simulink model "t_t_200_tge5"  (Simulink 6.2)
settings: Solver=ode45  StartTime=0.0  StopTime=10  RelTol=1e-3
undefined symbols (not defined in the file): BEE2_usr
libraries: xbsIndex_r3 x575, xps_library x48, casper_library x20
(part 1 of 4)
settings Model: LastModifiedBy=lspitler
settings DebuggingCC: SolverPrmCheckMsg=warning

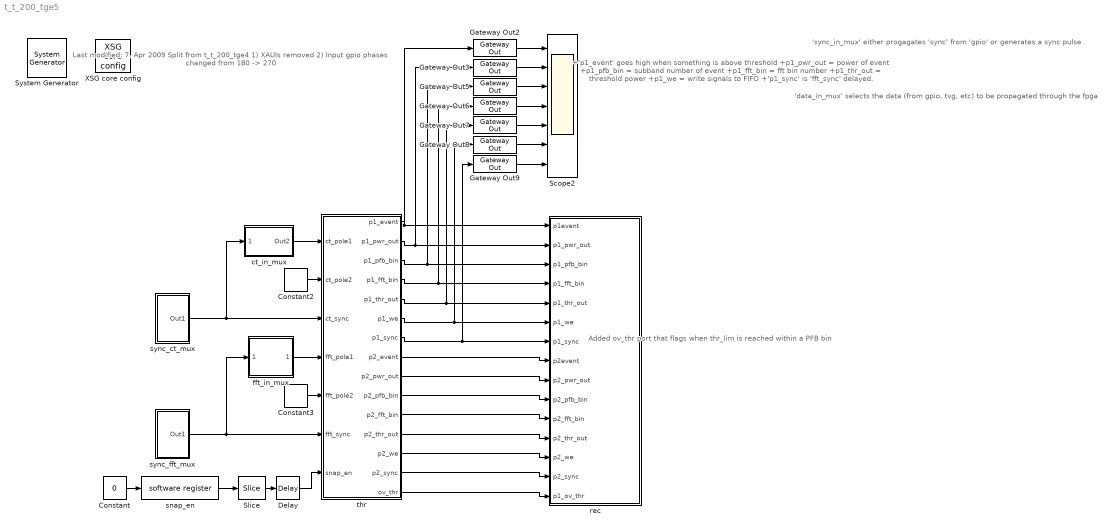
== system t_t_200_tge5 ==
  note: 'data_in_mux' selects
      | the data (from gpio, tvg, etc)
      | to be propagated
      | through the fpga
  note: 'sync_in_mux' either
      | progagates 'sync' from 'gpio'
      | or generates a sync pulse
  note: Last modified: 7. Apr 2009
      | Split from t_t_200_tge4
      | 1) XAUIs removed
      | 2) Input gpio phases changed
      | from 180 -> 270
  note: +'p1_event' goes high when something is above threshold
      | +p1_pwr_out = power of event
      | +p1_pfb_bin = subband number of event
      | +p1_fft_bin = fft bin number
      | +p1_thr_out = threshold power
      | +p1_we = write signals to FIFO
      | +'p1_sync' is 'fft_sync' delayed.
  note: Added ov_thr port that
      | flags when thr_lim is reached
      | within a PFB  bin
  " System Generator" : xbsIndex_r3/ System Generator  Tag=genX  xilinxfamily=Virtex2P  part=xc2vp70  speed=-7  package=ff1704  synthesis_tool=XST  directory=./t_t_200_tge5/sysgen  testbench=off  simulink_period=1  sysclk_period=5  incr_netlist=off  trim_vbits=Everywhere in SubSystem  dbl_ovrd=According to Block Masks  core_generation=According to Block Masks  run_coregen=off  deprecated_control=off  eval_field=0
      settings: AttributesFormatString=System\nGenerator
  Constant : Constant  Value=0
  Constant2 : xbsIndex_r3/Constant  const=0  equ=P=C  arith_type=Unsigned  n_bits=36  bin_pt=0  opselect=C  inp2=PCIN>>17  opr=+  inp1=P  carry=CIN  iostate=0  explicit_period=on  period=1  dbl_ovrd=off
  Constant3 : xbsIndex_r3/Constant  const=0  equ=P=C  arith_type=Unsigned  n_bits=36  bin_pt=0  opselect=C  inp2=PCIN>>17  opr=+  inp1=P  carry=CIN  iostate=0  explicit_period=on  period=1  dbl_ovrd=off
  Delay : xbsIndex_r3/Delay  latency=1  reg_retiming=on  explicit_period=off  period=1  en=off  accept_only_valid=off  init_zero=on  dbl_ovrd=off  show_param=off
      settings: xl_area=[0, 0, 0, 0, 0, 0, 0]
  Gateway Out{2..3,5..9} (7 alike) : xbsIndex_r3/Gateway Out  output_type=Double  nbits=8  bin_pt=6  arith_type=Boolean  quantization=Truncate  overflow=Wrap  hdl_port=on  timing_constraint=None  locs_specified=off  LOCs={}  needs_fixed_name=off  show_param=off
      settings: xl_area=[0, 0, 0, 0, 0, 0, 0]
  Scope2 : Scope  NumInputPorts=7
      settings: YMin=0.95~1.71474~-1~200~-1~0~-1  YMax=1.05~1.89524~1~900~1~1~1  SaveName=ScopeData21
  Slice : xbsIndex_r3/Slice  mode=Lower Bit Location + Width  nbits=1  bit1=0  base1=MSB of Input  bit0=0  base0=LSB of Input  boolean_output=on  explicit_period=off  period=1  dbl_ovrd=off
  XSG core config : xps_library/XSG core config  Tag=xps:xsg  hw_sys=BEE2_usr  ibob_linux=off  clk_src=usr_clk2x  gpio_clk_io_group=iBOB:sma  gpio_clk_bit_index=0  clk_rate=200  sample_period=1  synthesis_tool=XST  mpc_type=powerpc405
  ct_in_mux : Subsystem  mask{data_sel=3}
      mask prompts: data_sel "Data mux (0 = previous fpga, 1 = ones, 2 = zeros, 3 = tvg)"
  fft_in_mux : Subsystem  mask{data_sel=1}
      mask prompts: data_sel "Data mux (0 = previous fpga, 1 = tvg)"
  rec : Subsystem  mask{PFBSize=12, FFTSize=15, CPUWidth=32}
      mask prompts: PFBSize "PFB Size (2^?)"; FFTSize "FFT Size (2^?)"; CPUWidth "CPU Word Size"
  snap_en : xps_library/software register  Tag=xps:sw_reg  io_dir=From Processor  arith_type=Unsigned  bitwidth=32  bin_pt=0  sample_period=1  gw_name=t_t_200_tge5_snap_en_user_data_out
  sync_ct_mux : Subsystem  mask{sync_sel=1, sync_period=(2^18)-2}
      mask prompts: sync_sel "Sync Mux (0 = from previous FPGA, 1 = simulated sync)"; sync_period "Simulated sync period(number of clock cycles)"
  sync_fft_mux : Subsystem  mask{sync_sel=1, sync_period=(2^15)-2}
      mask prompts: sync_sel "Sync Mux (0 = from previous FPGA, 1 = simulated sync)"; sync_period "Simulated sync period(number of clock cycles)"
  thr : Subsystem  mask{PFBSize=12, FFTSize=15, DataWidth=18, CPUWidth=32}
      mask prompts: PFBSize "PFB Size (2^?)"; FFTSize "FFT Size (2^?)"; DataWidth "Data Bitwidth"; CPUWidth "CPU Word Size"
  wires:
  sync_ct_mux/1(Out1) -> ct_in_mux/1(trig_in), thr/3(ct_sync)
  Constant2/1 -> thr/2(ct_pole2)
  Constant3/1 -> thr/5(fft_pole2)
  thr/2(p1_pwr_out) -> Gateway Out3/1, rec/2(p1_pwr_out)
  thr/3(p1_pfb_bin) -> Gateway Out5/1, rec/3(p1_pfb_bin)
  thr/4(p1_fft_bin) -> Gateway Out6/1, rec/4(p1_fft_bin)
  thr/5(p1_thr_out) -> Gateway Out7/1, rec/5(p1_thr_out)
  thr/1(p1_event) -> Gateway Out2/1, rec/1(p1event)
  Gateway Out2/1 -> Scope2/1
  Gateway Out3/1 -> Scope2/2
  Gateway Out5/1 -> Scope2/3
  Gateway Out6/1 -> Scope2/4
  Gateway Out7/1 -> Scope2/5
  Gateway Out8/1 -> Scope2/6
  Gateway Out9/1 -> Scope2/7
  thr/6(p1_we) -> Gateway Out8/1, rec/6(p1_we)
  thr/7(p1_sync) -> Gateway Out9/1, rec/7(p1_sync)
  Constant/1 -> snap_en/1
  snap_en/1 -> Slice/1
  Slice/1 -> Delay/1
  thr/8(p2_event) -> rec/8(p2event)
  thr/9(p2_pwr_out) -> rec/9(p2_pwr_out)
  thr/10(p2_pfb_bin) -> rec/10(p2_pfb_bin)
  thr/11(p2_fft_bin) -> rec/11(p2_fft_bin)
  thr/12(p2_thr_out) -> rec/12(p2_thr_out)
  thr/13(p2_we) -> rec/13(p2_we)
  thr/14(p2_sync) -> rec/14(p2_sync)
  thr/15(ov_thr) -> rec/15(p1_ov_thr)
  sync_fft_mux/1(Out1) -> fft_in_mux/1(trig_in), thr/6(fft_sync)
  ct_in_mux/1(Out2) -> thr/1(ct_pole1)
  fft_in_mux/1(Out2) -> thr/4(fft_pole1)
  Delay/1 -> thr/7("snap_en ")

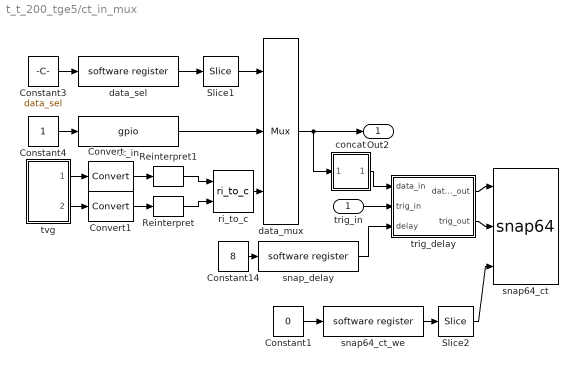
== system t_t_200_tge5/ct_in_mux ==
  trig_in : Inport  Port=1  LatchInput=off
  Constant1 : Constant  Value=0
  Constant14 : Constant  Value=8
  Constant3 : Constant  Value=data_sel
  Constant4 : Constant
  Convert : xbsIndex_r3/Convert  arith_type=Unsigned  n_bits=18  bin_pt=0  quantization=Truncate  overflow=Wrap  latency=0  explicit_period=on  period=1  dbl_ovrd=off  show_param=off  inserted_by_tool=off  pipeline=off
      settings: xl_area=[0, 0, 0, 0, 0, 0, 0]
  Convert1 : xbsIndex_r3/Convert  arith_type=Unsigned  n_bits=18  bin_pt=0  quantization=Truncate  overflow=Wrap  latency=0  explicit_period=on  period=1  dbl_ovrd=off  show_param=off  inserted_by_tool=off  pipeline=off
      settings: xl_area=[0, 0, 0, 0, 0, 0, 0]
  Reinterpret : xbsIndex_r3/Reinterpret  force_arith_type=on  arith_type="Signed  (2's comp)"  force_bin_pt=on  bin_pt=17  force_valid=on
  Reinterpret1 : xbsIndex_r3/Reinterpret  force_arith_type=on  arith_type="Signed  (2's comp)"  force_bin_pt=on  bin_pt=17  force_valid=on
  Slice1 : xbsIndex_r3/Slice  mode=Lower Bit Location + Width  nbits=1  bit1=0  base1=MSB of Input  bit0=0  base0=LSB of Input  boolean_output=off  explicit_period=off  period=1  dbl_ovrd=off
  Slice2 : xbsIndex_r3/Slice  mode=Lower Bit Location + Width  nbits=1  bit1=0  base1=MSB of Input  bit0=0  base0=LSB of Input  boolean_output=on  explicit_period=off  period=1  dbl_ovrd=off
  concat : Subsystem
  ct_in : xps_library/gpio  Tag=xps:gpio  io_group=BEE2_usr:rightlink  io_dir=in  arith_type=Unsigned  bitwidth=36  bin_pt=0  bit_index=[0:35]  sample_period=1  use_single_ended=off  use_ddr=off  reg_iob=on  reg_clk_phase=270  termination=None
  data_mux : xbsIndex_r3/Mux  inputs=2  precision=Full  arith_type="Signed  (2's comp)"  n_bits=8  bin_pt=2  quantization=Truncate  overflow=Wrap  latency=2  explicit_period=on  period=1  en=off  dbl_ovrd=off  show_param=off  mux_type=off  use_rpm=off  gen_core=off
      settings: xl_area=[0, 0, 0, 0, 0, 0, 0]
  data_sel : xps_library/software register  Tag=xps:sw_reg  io_dir=From Processor  arith_type=Unsigned  bitwidth=32  bin_pt=0  sample_period=1  gw_name=t_t_200_tge5_ct_in_mux_data_sel_user_data_out
  ri_to_c : casper_library/Misc/ri_to_c
  snap64_ct : casper_library/Scopes/snap64  nsamples=11
  snap64_ct_we : xps_library/software register  Tag=xps:sw_reg  io_dir=From Processor  arith_type=Unsigned  bitwidth=32  bin_pt=0  sample_period=1  gw_name=t_t_200_tge5_ct_in_mux_snap64_ct_we_user_data_out
  snap_delay : xps_library/software register  Tag=xps:sw_reg  io_dir=From Processor  arith_type=Unsigned  bitwidth=32  bin_pt=0  sample_period=1  gw_name=t_t_200_tge5_ct_in_mux_snap_delay_user_data_out
  trig_delay : Subsystem
  tvg : Subsystem
  Out2 : Outport
  wires:
  data_sel/1 -> Slice1/1
  Constant3/1 -> data_sel/1
  Slice1/1 -> data_mux/1
  ct_in/1 -> data_mux/2
  Constant4/1 -> ct_in/1
  data_mux/1 -> Out2/1, concat/1(In1)
  ri_to_c/1 -> data_mux/3
  Convert/1 -> Reinterpret1/1
  Convert1/1 -> Reinterpret/1
  Reinterpret1/1 -> ri_to_c/1
  Reinterpret/1 -> ri_to_c/2
  tvg/1(re_out) -> Convert/1
  tvg/2(im_out) -> Convert1/1
  Constant1/1 -> snap64_ct_we/1
  snap64_ct_we/1 -> Slice2/1
  Slice2/1 -> snap64_ct/3
  Constant14/1 -> snap_delay/1
  snap_delay/1 -> trig_delay/3(delay)
  trig_delay/1(data_out) -> snap64_ct/1
  trig_delay/2(trig_out) -> snap64_ct/2
  concat/1(Out1) -> trig_delay/1(data_in)
  trig_in/1 -> trig_delay/2(trig_in)

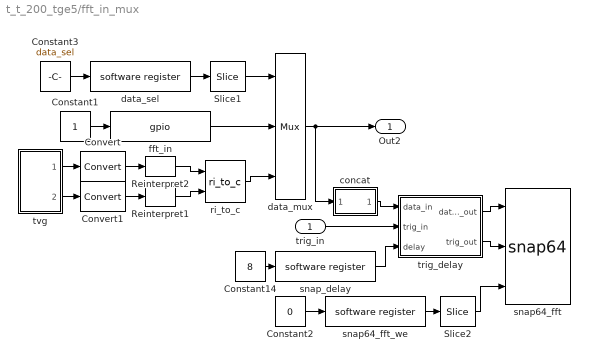
== system t_t_200_tge5/fft_in_mux ==
  trig_in : Inport  Port=1  LatchInput=off
  Constant1 : Constant
  Constant14 : Constant  Value=8
  Constant2 : Constant  Value=0
  Constant3 : Constant  Value=data_sel
  Convert : xbsIndex_r3/Convert  arith_type=Unsigned  n_bits=18  bin_pt=0  quantization=Truncate  overflow=Wrap  latency=0  explicit_period=on  period=1  dbl_ovrd=off  show_param=off  inserted_by_tool=off  pipeline=off
      settings: xl_area=[0, 0, 0, 0, 0, 0, 0]
  Convert1 : xbsIndex_r3/Convert  arith_type=Unsigned  n_bits=18  bin_pt=0  quantization=Truncate  overflow=Wrap  latency=0  explicit_period=on  period=1  dbl_ovrd=off  show_param=off  inserted_by_tool=off  pipeline=off
      settings: xl_area=[0, 0, 0, 0, 0, 0, 0]
  Reinterpret1 : xbsIndex_r3/Reinterpret  force_arith_type=on  arith_type="Signed  (2's comp)"  force_bin_pt=on  bin_pt=17  force_valid=on
  Reinterpret2 : xbsIndex_r3/Reinterpret  force_arith_type=on  arith_type="Signed  (2's comp)"  force_bin_pt=on  bin_pt=17  force_valid=on
  Slice1 : xbsIndex_r3/Slice  mode=Lower Bit Location + Width  nbits=1  bit1=0  base1=MSB of Input  bit0=0  base0=LSB of Input  boolean_output=off  explicit_period=off  period=1  dbl_ovrd=off
  Slice2 : xbsIndex_r3/Slice  mode=Lower Bit Location + Width  nbits=1  bit1=0  base1=MSB of Input  bit0=0  base0=LSB of Input  boolean_output=on  explicit_period=off  period=1  dbl_ovrd=off
  concat : Subsystem
  data_mux : xbsIndex_r3/Mux  inputs=2  precision=Full  arith_type="Signed  (2's comp)"  n_bits=8  bin_pt=2  quantization=Truncate  overflow=Wrap  latency=2  explicit_period=on  period=1  en=off  dbl_ovrd=off  show_param=off  mux_type=off  use_rpm=off  gen_core=off
      settings: xl_area=[0, 0, 0, 0, 0, 0, 0]
  data_sel : xps_library/software register  Tag=xps:sw_reg  io_dir=From Processor  arith_type=Unsigned  bitwidth=32  bin_pt=0  sample_period=1  gw_name=t_t_200_tge5_fft_in_mux_data_sel_user_data_out
  fft_in : xps_library/gpio  Tag=xps:gpio  io_group=BEE2_usr:rightlink  io_dir=in  arith_type=Unsigned  bitwidth=36  bin_pt=0  bit_index=[37:72]  sample_period=1  use_single_ended=off  use_ddr=off  reg_iob=on  reg_clk_phase=270  termination=None
  ri_to_c : casper_library/Misc/ri_to_c
  snap64_fft : casper_library/Scopes/snap64  nsamples=11
  snap64_fft_we : xps_library/software register  Tag=xps:sw_reg  io_dir=From Processor  arith_type=Unsigned  bitwidth=32  bin_pt=0  sample_period=1  gw_name=t_t_200_tge5_fft_in_mux_snap64_fft_we_user_data_out
  snap_delay : xps_library/software register  Tag=xps:sw_reg  io_dir=From Processor  arith_type=Unsigned  bitwidth=32  bin_pt=0  sample_period=1  gw_name=t_t_200_tge5_fft_in_mux_snap_delay_user_data_out
  trig_delay : Subsystem
  tvg : Subsystem
  Out2 : Outport
  wires:
  data_sel/1 -> Slice1/1
  Constant3/1 -> data_sel/1
  Slice1/1 -> data_mux/1
  fft_in/1 -> data_mux/2
  Constant1/1 -> fft_in/1
  data_mux/1 -> Out2/1, concat/1(In1)
  Convert1/1 -> Reinterpret1/1
  Reinterpret1/1 -> ri_to_c/2
  tvg/2(im_out) -> Convert1/1
  tvg/1(re_out) -> Convert/1
  Convert/1 -> Reinterpret2/1
  Reinterpret2/1 -> ri_to_c/1
  ri_to_c/1 -> data_mux/3
  Constant2/1 -> snap64_fft_we/1
  snap64_fft_we/1 -> Slice2/1
  Slice2/1 -> snap64_fft/3
  Constant14/1 -> snap_delay/1
  snap_delay/1 -> trig_delay/3(delay)
  trig_delay/1(data_out) -> snap64_fft/1
  trig_delay/2(trig_out) -> snap64_fft/2
  concat/1(Out1) -> trig_delay/1(data_in)
  trig_in/1 -> trig_delay/2(trig_in)

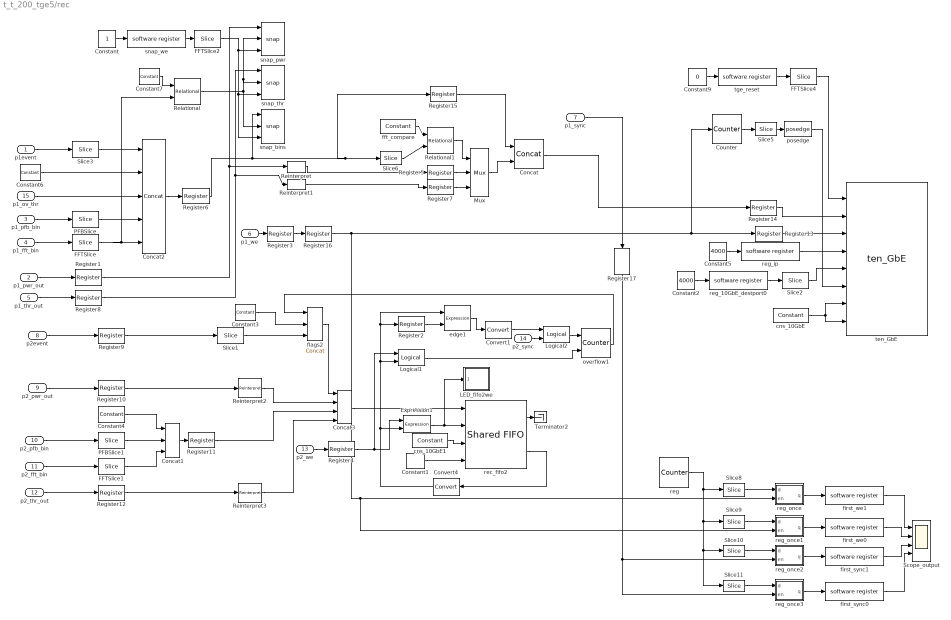
== system t_t_200_tge5/rec ==
  p1event : Inport  Port=1  LatchInput=off
  p1_pwr_out : Inport  Port=2  LatchInput=off
  p1_pfb_bin : Inport  Port=3  LatchInput=off
  p1_fft_bin : Inport  Port=4  LatchInput=off
  p1_thr_out : Inport  Port=5  LatchInput=off
  p1_we : Inport  Port=6  LatchInput=off
  p1_sync : Inport  Port=7  LatchInput=off
  p2event : Inport  Port=8  LatchInput=off
  p2_pwr_out : Inport  Port=9  LatchInput=off
  p2_pfb_bin : Inport  Port=10  LatchInput=off
  p2_fft_bin : Inport  Port=11  LatchInput=off
  p2_thr_out : Inport  Port=12  LatchInput=off
  p2_we : Inport  Port=13  LatchInput=off
  p2_sync : Inport  Port=14  LatchInput=off
  p1_ov_thr : Inport  Port=15  LatchInput=off
  Concat : xbsIndex_r3/Concat  num_inputs=2  explicit_period=off  period=1  dbl_ovrd=off
  Concat1 : xbsIndex_r3/Concat  num_inputs=3  explicit_period=off  period=1  dbl_ovrd=off
  Concat2 : xbsIndex_r3/Concat  num_inputs=5  explicit_period=on  period=1  dbl_ovrd=off
  Concat3 : xbsIndex_r3/Concat  num_inputs=4  explicit_period=off  period=1  dbl_ovrd=off
  Constant : Constant
  Constant1 : xbsIndex_r3/Constant  const=512-4  equ=P=C  arith_type=Unsigned  n_bits=32  bin_pt=0  opselect=C  inp2=PCIN>>17  opr=+  inp1=P  carry=CIN  iostate=0  explicit_period=on  period=1  dbl_ovrd=off
  Constant2 : Constant  Value=4000
  Constant3 : xbsIndex_r3/Constant  const=0  equ=P=C  arith_type=Unsigned  n_bits=15  bin_pt=0  opselect=C  inp2=PCIN>>17  opr=+  inp1=P  carry=CIN  iostate=0  explicit_period=on  period=1  dbl_ovrd=off
  Constant4 : xbsIndex_r3/Constant  const=0  equ=P=C  arith_type=Unsigned  n_bits=CPUWidth-PFBSize-FFTSize  bin_pt=0  opselect=C  inp2=PCIN>>17  opr=+  inp1=P  carry=CIN  iostate=0  explicit_period=on  period=1  dbl_ovrd=off
  Constant5 : Constant  Value=4000
  Constant6 : xbsIndex_r3/Constant  const=0  equ=P=C  arith_type=Unsigned  n_bits=3  bin_pt=0  opselect=C  inp2=PCIN>>17  opr=+  inp1=P  carry=CIN  iostate=0  explicit_period=on  period=1  dbl_ovrd=off
  Constant7 : xbsIndex_r3/Constant  const=0  equ=P=C  arith_type=Unsigned  n_bits=15  bin_pt=0  opselect=C  inp2=PCIN>>17  opr=+  inp1=P  carry=CIN  iostate=0  explicit_period=on  period=1  dbl_ovrd=off
  Constant9 : Constant  Value=0
  Convert1 : xbsIndex_r3/Convert  arith_type=Boolean  n_bits=8  bin_pt=6  quantization=Truncate  overflow=Wrap  latency=0  explicit_period=off  period=1  dbl_ovrd=off  show_param=off  inserted_by_tool=off  pipeline=off
      settings: xl_area=[0, 0, 0, 0, 0, 0, 0]
  Convert4 : xbsIndex_r3/Convert  Orientation=left  arith_type=Boolean  n_bits=8  bin_pt=6  quantization=Truncate  overflow=Wrap  latency=0  explicit_period=off  period=1  dbl_ovrd=off  show_param=off  inserted_by_tool=off  pipeline=off
      settings: xl_area=[0, 0, 0, 0, 0, 0, 0]
  Counter : xbsIndex_r3/Counter  cnt_type=Free Running  n_bits=9  bin_pt=0  arith_type=Unsigned  start_count=0  cnt_to=Inf  cnt_by_val=1  operation=Up  explicit_period=off  period=1  load_pin=off  rst=off  en=on  dbl_ovrd=off  show_param=off  use_rpm=on  gen_core=off
      settings: xl_area=[0, 0, 0, 0, 0, 0, 0]
  Expression1 : xbsIndex_r3/Expression  expression=a & ~b  precision=Full  arith_type=Unsigned  n_bits=8  bin_pt=2  align_bp=on  latency=0  explicit_period=off  period=1  en=off  dbl_ovrd=off  show_param=off
      settings: xl_area=[0, 0, 0, 0, 0, 0, 0]
  FFTSlice : xbsIndex_r3/Slice  mode=Lower Bit Location + Width  nbits=FFTSize  bit1=0  base1=MSB of Input  bit0=0  base0=LSB of Input  boolean_output=off  explicit_period=off  period=1  dbl_ovrd=off
  FFTSlice1 : xbsIndex_r3/Slice  mode=Lower Bit Location + Width  nbits=FFTSize  bit1=0  base1=MSB of Input  bit0=0  base0=LSB of Input  boolean_output=off  explicit_period=off  period=1  dbl_ovrd=off
  FFTSlice2 : xbsIndex_r3/Slice  mode=Lower Bit Location + Width  nbits=1  bit1=0  base1=MSB of Input  bit0=0  base0=LSB of Input  boolean_output=on  explicit_period=off  period=1  dbl_ovrd=off
  FFTSlice4 : xbsIndex_r3/Slice  mode=Lower Bit Location + Width  nbits=1  bit1=0  base1=MSB of Input  bit0=0  base0=LSB of Input  boolean_output=on  explicit_period=off  period=1  dbl_ovrd=off
  LED_fifo2we : Subsystem  mask{pulse_length=200000}
      mask prompts: pulse_length "Pulse Length (samples)"
  Logical1 : xbsIndex_r3/Logical  logical_function=AND  inputs=2  precision=Full  arith_type=Unsigned  n_bits=8  bin_pt=2  align_bp=on  latency=0  explicit_period=off  period=1  en=off  dbl_ovrd=off  show_param=off
      settings: xl_area=[0, 0, 0, 0, 0, 0, 0]
  Logical2 : xbsIndex_r3/Logical  logical_function=OR  inputs=2  precision=Full  arith_type=Unsigned  n_bits=8  bin_pt=2  align_bp=on  latency=0  explicit_period=off  period=1  en=off  dbl_ovrd=off  show_param=off
      settings: xl_area=[0, 0, 0, 0, 0, 0, 0]
  Mux : xbsIndex_r3/Mux  inputs=2  precision=Full  arith_type="Signed  (2's comp)"  n_bits=8  bin_pt=2  quantization=Truncate  overflow=Wrap  latency=0  explicit_period=off  period=1  en=off  dbl_ovrd=off  show_param=off  mux_type=off  use_rpm=off  gen_core=off
      settings: xl_area=[0, 0, 0, 0, 0, 0, 0]
  PFBSlice : xbsIndex_r3/Slice  mode=Lower Bit Location + Width  nbits=PFBSize  bit1=0  base1=MSB of Input  bit0=0  base0=LSB of Input  boolean_output=off  explicit_period=off  period=1  dbl_ovrd=off
  PFBSlice1 : xbsIndex_r3/Slice  mode=Lower Bit Location + Width  nbits=PFBSize  bit1=0  base1=MSB of Input  bit0=0  base0=LSB of Input  boolean_output=off  explicit_period=off  period=1  dbl_ovrd=off
  Register{1..16} (16 alike) : xbsIndex_r3/Register  init=0  reg_only_valid=off  explicit_period=on  period=1  rst=off  en=off  out_en=off  dbl_ovrd=off  show_param=off
      settings: xl_area=[0, 0, 0, 0, 0, 0, 0]
  Register17 : xbsIndex_r3/Register  Orientation=down  init=0  reg_only_valid=off  explicit_period=on  period=1  rst=off  en=off  out_en=off  dbl_ovrd=off  show_param=off
      settings: xl_area=[0, 0, 0, 0, 0, 0, 0]
  Reinterpret{,1..3} (4 alike) : xbsIndex_r3/Reinterpret  force_arith_type=on  arith_type=Unsigned  force_bin_pt=on  bin_pt=0  force_valid=on
  Relational : xbsIndex_r3/Relational  mode=a=b  latency=1  explicit_period=off  period=1  en=off  dbl_ovrd=off  show_param=off
      settings: xl_area=[0, 0, 0, 0, 0, 0, 0]
  Relational1 : xbsIndex_r3/Relational  mode=a=b  latency=1  explicit_period=off  period=1  en=off  dbl_ovrd=off  show_param=off
      settings: xl_area=[0, 0, 0, 0, 0, 0, 0]
  Scope_output : Scope  NumInputPorts=4
      settings: TimeRange=1  YMin=502.55~502.55~500.65~500.65  YMax=555.45~555.45~553.35~553.35  SaveName=ScopeData5
  Slice1 : xbsIndex_r3/Slice  mode=Lower Bit Location + Width  nbits=1  bit1=0  base1=MSB of Input  bit0=0  base0=LSB of Input  boolean_output=off  explicit_period=off  period=1  dbl_ovrd=off
  Slice10 : xbsIndex_r3/Slice  mode=Upper Bit Location + Width  nbits=32  bit1=0  base1=MSB of Input  bit0=0  base0=LSB of Input  boolean_output=off  explicit_period=off  period=1  dbl_ovrd=off
  Slice11 : xbsIndex_r3/Slice  mode=Lower Bit Location + Width  nbits=32  bit1=-3  base1=MSB of Input  bit0=0  base0=LSB of Input  boolean_output=off  explicit_period=off  period=1  dbl_ovrd=off
  Slice2 : xbsIndex_r3/Slice  mode=Lower Bit Location + Width  nbits=16  bit1=0  base1=MSB of Input  bit0=0  base0=LSB of Input  boolean_output=off  explicit_period=off  period=1  dbl_ovrd=off
  Slice3 : xbsIndex_r3/Slice  mode=Lower Bit Location + Width  nbits=1  bit1=0  base1=MSB of Input  bit0=0  base0=LSB of Input  boolean_output=off  explicit_period=off  period=1  dbl_ovrd=off
  Slice5 : xbsIndex_r3/Slice  mode=Upper Bit Location + Width  nbits=1  bit1=0  base1=MSB of Input  bit0=64  base0=LSB of Input  boolean_output=on  explicit_period=off  period=1  dbl_ovrd=off
  Slice6 : xbsIndex_r3/Slice  mode=Lower Bit Location + Width  nbits=15  bit1=0  base1=MSB of Input  bit0=0  base0=LSB of Input  boolean_output=off  explicit_period=off  period=1  dbl_ovrd=off
  Slice8 : xbsIndex_r3/Slice  mode=Upper Bit Location + Width  nbits=32  bit1=0  base1=MSB of Input  bit0=0  base0=LSB of Input  boolean_output=off  explicit_period=off  period=1  dbl_ovrd=off
  Slice9 : xbsIndex_r3/Slice  mode=Lower Bit Location + Width  nbits=32  bit1=-3  base1=MSB of Input  bit0=0  base0=LSB of Input  boolean_output=off  explicit_period=off  period=1  dbl_ovrd=off
  Terminator2 : Terminator
  cns_10GbE : xbsIndex_r3/Constant  const=0  equ=P=C  arith_type=Boolean  n_bits=32  bin_pt=0  opselect=C  inp2=PCIN>>17  opr=+  inp1=P  carry=CIN  iostate=0  explicit_period=on  period=1  dbl_ovrd=off
  cns_10GbE1 : xbsIndex_r3/Constant  const=0  equ=P=C  arith_type=Boolean  n_bits=32  bin_pt=0  opselect=C  inp2=PCIN>>17  opr=+  inp1=P  carry=CIN  iostate=0  explicit_period=on  period=1  dbl_ovrd=off
  edge1 : xbsIndex_r3/Expression  expression=a & ~b  precision=Full  arith_type=Unsigned  n_bits=8  bin_pt=2  align_bp=on  latency=0  explicit_period=off  period=1  en=off  dbl_ovrd=off  show_param=off
      settings: xl_area=[0, 0, 0, 0, 0, 0, 0]
  fft_compare : xbsIndex_r3/Constant  const=0  equ=P=C  arith_type=Unsigned  n_bits=15  bin_pt=0  opselect=C  inp2=PCIN>>17  opr=+  inp1=P  carry=CIN  iostate=0  explicit_period=on  period=1  dbl_ovrd=off
  first_sync0 : xps_library/software register  Tag=xps:sw_reg  io_dir=To Processor  arith_type=Unsigned  bitwidth=32  bin_pt=0  sample_period=1  gw_name=t_t_200_tge5_rec_first_sync0_user_data_in
  first_sync1 : xps_library/software register  Tag=xps:sw_reg  io_dir=To Processor  arith_type=Unsigned  bitwidth=32  bin_pt=0  sample_period=1  gw_name=t_t_200_tge5_rec_first_sync1_user_data_in
  first_we0 : xps_library/software register  Tag=xps:sw_reg  io_dir=To Processor  arith_type=Unsigned  bitwidth=32  bin_pt=0  sample_period=1  gw_name=t_t_200_tge5_rec_first_we0_user_data_in
  first_we1 : xps_library/software register  Tag=xps:sw_reg  io_dir=To Processor  arith_type=Unsigned  bitwidth=32  bin_pt=0  sample_period=1  gw_name=t_t_200_tge5_rec_first_we1_user_data_in
  flags2 : xbsIndex_r3/Concat  num_inputs=3  explicit_period=off  period=1  dbl_ovrd=off
  overflow1 : xbsIndex_r3/Counter  cnt_type=Count Limited  n_bits=16  bin_pt=0  arith_type=Unsigned  start_count=0  cnt_to=Inf  cnt_by_val=1  operation=Up  explicit_period=off  period=1  load_pin=off  rst=on  en=on  dbl_ovrd=off  show_param=off  use_rpm=on  gen_core=off
      settings: xl_area=[0, 0, 0, 0, 0, 0, 0]
  posedge : casper_library/Misc/posedge  Tag=Rising Edge Detector
  rec_fifo2 : xps_library/Shared FIFO  Tag=xps:fifo  io_dir=To Processor  arith_type=Unsigned  data_width=128  data_bin_pt=0  fifo_length=512
  reg : xbsIndex_r3/Counter  cnt_type=Free Running  n_bits=64  bin_pt=0  arith_type=Unsigned  start_count=0  cnt_to=Inf  cnt_by_val=1  operation=Up  explicit_period=off  period=1  load_pin=off  rst=off  en=off  dbl_ovrd=off  show_param=off  use_rpm=on  gen_core=off
      settings: xl_area=[0, 0, 0, 0, 0, 0, 0]
  reg_10GbE_destport0 : xps_library/software register  Tag=xps:sw_reg  io_dir=From Processor  arith_type=Unsigned  bitwidth=32  bin_pt=0  sample_period=1  gw_name=t_t_200_tge5_rec_reg_10GbE_destport0_user_data_out
  reg_ip : xps_library/software register  Tag=xps:sw_reg  io_dir=From Processor  arith_type=Unsigned  bitwidth=32  bin_pt=0  sample_period=1  gw_name=t_t_200_tge5_rec_reg_ip_user_data_out
  reg_once : Subsystem
  reg_once1 : Subsystem
  reg_once2 : Subsystem
  reg_once3 : Subsystem
  snap_bins : casper_library/Scopes/snap  nsamples=12
  snap_pwr : casper_library/Scopes/snap  nsamples=12
  snap_thr : casper_library/Scopes/snap  nsamples=12
  snap_we : xps_library/software register  Tag=xps:sw_reg  io_dir=From Processor  arith_type=Unsigned  bitwidth=32  bin_pt=0  sample_period=1  gw_name=t_t_200_tge5_rec_snap_we_user_data_out
  ten_GbE : xps_library/ten_GbE  Tag=xps:tengbe  port=BEE2_usr:3  mac_lite=off  show_param=on  pre_emph=3  swing=800
  tge_reset : xps_library/software register  Tag=xps:sw_reg  io_dir=From Processor  arith_type=Unsigned  bitwidth=32  bin_pt=0  sample_period=1  gw_name=t_t_200_tge5_rec_tge_reset_user_data_out
  wires:
  first_we1/1 -> Scope_output/1
  first_sync0/1 -> Scope_output/4
  first_sync1/1 -> Scope_output/3
  first_we0/1 -> Scope_output/2
  reg_once3/1(q) -> first_sync0/1
  Slice11/1 -> reg_once3/1(d)
  reg_once2/1(q) -> first_sync1/1
  Slice10/1 -> reg_once2/1(d)
  reg_once1/1(q) -> first_we0/1
  Slice9/1 -> reg_once1/1(d)
  reg_once/1(q) -> first_we1/1
  Slice8/1 -> reg_once/1(d)
  reg/1 -> Slice11/1, Slice10/1, Slice9/1, Slice8/1
  Register4/1 -> Expression1/1, Logical1/1
  Register3/1 -> Register16/1
  Convert4/1 -> Logical1/2, Register2/1, edge1/1, Expression1/2
  Convert1/1 -> Logical2/1
  Reinterpret3/1 -> Concat3/4
  Reinterpret2/1 -> Concat3/2
  Reinterpret1/1 -> Register7/1
  Concat3/1 -> rec_fifo2/1
  Register12/1 -> Reinterpret3/1
  Register11/1 -> Concat3/3
  Register10/1 -> Reinterpret2/1
  p2_thr_out/1 -> Register12/1
  p2_pwr_out/1 -> Register10/1
  p2_fft_bin/1 -> FFTSlice1/1
  FFTSlice1/1 -> Concat1/3
  PFBSlice1/1 -> Concat1/2
  Constant4/1 -> Concat1/1
  Concat1/1 -> Register11/1
  p2_pfb_bin/1 -> PFBSlice1/1
  Logical1/1 -> overflow1/2
  Logical2/1 -> overflow1/1
  edge1/1 -> Convert1/1
  Register9/1 -> Slice1/1
  Constant3/1 -> flags2/2
  flags2/1 -> Concat3/1
  Slice1/1 -> flags2/3
  overflow1/1 -> flags2/1
  Register2/1 -> edge1/2
  p2_sync/1 -> Logical2/2
  p2event/1 -> Register9/1
  rec_fifo2/1 -> Terminator2/1
  Constant1/1 -> rec_fifo2/4
  rec_fifo2/2 -> Convert4/1
  p2_we/1 -> Register4/1
  Expression1/1 -> LED_fifo2we/1(Sync_In), rec_fifo2/2
  Register8/1 -> Reinterpret1/1, snap_thr/1
  Register1/1 -> snap_pwr/1, Reinterpret/1
  p1_thr_out/1 -> Register8/1
  p1_pwr_out/1 -> Register1/1
  p1_fft_bin/1 -> FFTSlice/1
  Concat2/1 -> Register6/1
  p1_pfb_bin/1 -> PFBSlice/1
  p1_sync/1 -> Register17/1
  p1_we/1 -> Register3/1
  Register6/1 -> snap_bins/1, Slice6/1, Register15/1
  Reinterpret/1 -> Register5/1
  Constant6/1 -> Concat2/2
  Slice3/1 -> Concat2/1
  snap_we/1 -> FFTSlice2/1
  Constant/1 -> snap_we/1
  FFTSlice2/1 -> snap_pwr/3, snap_thr/3, snap_bins/3
  p1event/1 -> Slice3/1
  Constant7/1 -> Relational/1
  Relational/1 -> snap_pwr/2, snap_thr/2, snap_bins/2
  FFTSlice/1 -> Concat2/5, Relational/2
  PFBSlice/1 -> Concat2/4
  p1_ov_thr/1 -> Concat2/3
  reg_10GbE_destport0/1 -> Slice2/1
  Constant2/1 -> reg_10GbE_destport0/1
  Slice2/1 -> ten_GbE/5
  Constant5/1 -> reg_ip/1
  reg_ip/1 -> ten_GbE/4
  cns_10GbE/1 -> ten_GbE/8, ten_GbE/7
  Constant9/1 -> tge_reset/1
  tge_reset/1 -> FFTSlice4/1
  FFTSlice4/1 -> ten_GbE/1
  Concat/1 -> Register14/1
  Slice5/1 -> posedge/1
  Counter/1 -> Slice5/1
  posedge/1 -> ten_GbE/6
  Register13/1 -> ten_GbE/3
  Register14/1 -> ten_GbE/2
  fft_compare/1 -> Relational1/1
  Slice6/1 -> Relational1/2
  Relational1/1 -> Mux/1
  Register5/1 -> Mux/2
  Register7/1 -> Mux/3
  cns_10GbE1/1 -> rec_fifo2/3
  Register15/1 -> Concat/1
  Mux/1 -> Concat/2
  Register16/1 -> reg_once1/2(en), reg_once/2(en), Counter/1, Register13/1
  Register17/1 -> reg_once3/2(en), reg_once2/2(en)

== system t_t_200_tge5/sync_ct_mux ==
  Constant : Constant  Value=sync_sel
  Constant1 : Constant
  Constant2 : Constant  Value=sync_period
  Constant3 : xbsIndex_r3/Constant  const=1  equ=P=C  arith_type=Unsigned  n_bits=32  bin_pt=0  opselect=C  inp2=PCIN>>17  opr=+  inp1=P  carry=CIN  iostate=0  explicit_period=on  period=1  dbl_ovrd=off
  Counter : xbsIndex_r3/Counter  cnt_type=Free Running  n_bits=32  bin_pt=0  arith_type=Unsigned  start_count=0  cnt_to=Inf  cnt_by_val=1  operation=Up  explicit_period=on  period=1  load_pin=on  rst=off  en=off  dbl_ovrd=off  show_param=off  use_rpm=on  gen_core=off
      settings: xl_area=[0, 0, 0, 0, 0, 0, 0]
  Relational : xbsIndex_r3/Relational  mode=a=b  latency=1  explicit_period=off  period=1  en=off  dbl_ovrd=off  show_param=off
      settings: xl_area=[0, 0, 0, 0, 0, 0, 0]
  Slice : xbsIndex_r3/Slice  mode=Lower Bit Location + Width  nbits=1  bit1=0  base1=MSB of Input  bit0=0  base0=LSB of Input  boolean_output=off  explicit_period=off  period=1  dbl_ovrd=off
  ctsync_in : xps_library/gpio  Tag=xps:gpio  io_group=BEE2_usr:rightlink  io_dir=in  arith_type=Boolean  bitwidth=1  bin_pt=0  bit_index=36  sample_period=1  use_single_ended=off  use_ddr=off  reg_iob=on  reg_clk_phase=270  termination=None
  sync_mux : xbsIndex_r3/Mux  inputs=2  precision=Full  arith_type="Signed  (2's comp)"  n_bits=8  bin_pt=2  quantization=Truncate  overflow=Wrap  latency=2  explicit_period=on  period=1  en=off  dbl_ovrd=off  show_param=off  mux_type=off  use_rpm=off  gen_core=off
      settings: xl_area=[0, 0, 0, 0, 0, 0, 0]
  sync_per : xps_library/software register  Tag=xps:sw_reg  io_dir=From Processor  arith_type=Unsigned  bitwidth=32  bin_pt=0  sample_period=1  gw_name=t_t_200_tge5_sync_ct_mux_sync_per_user_data_out
  sync_sel : xps_library/software register  Tag=xps:sw_reg  io_dir=From Processor  arith_type=Unsigned  bitwidth=32  bin_pt=0  sample_period=1  gw_name=t_t_200_tge5_sync_ct_mux_sync_sel_user_data_out
  Out1 : Outport
  wires:
  sync_sel/1 -> Slice/1
  Constant/1 -> sync_sel/1
  Constant1/1 -> ctsync_in/1
  Constant2/1 -> sync_per/1
  Slice/1 -> sync_mux/1
  ctsync_in/1 -> sync_mux/2
  Counter/1 -> Relational/2
  sync_per/1 -> Relational/1
  Relational/1 -> Counter/1, sync_mux/3
  sync_mux/1 -> Out1/1
  Constant3/1 -> Counter/2

== system t_t_200_tge5/sync_fft_mux ==
  Constant : Constant  Value=sync_sel
  Constant1 : Constant
  Constant2 : Constant  Value=sync_period
  Constant3 : xbsIndex_r3/Constant  const=1  equ=P=C  arith_type=Unsigned  n_bits=32  bin_pt=0  opselect=C  inp2=PCIN>>17  opr=+  inp1=P  carry=CIN  iostate=0  explicit_period=on  period=1  dbl_ovrd=off
  Counter : xbsIndex_r3/Counter  cnt_type=Free Running  n_bits=32  bin_pt=0  arith_type=Unsigned  start_count=0  cnt_to=Inf  cnt_by_val=1  operation=Up  explicit_period=on  period=1  load_pin=on  rst=off  en=off  dbl_ovrd=off  show_param=off  use_rpm=on  gen_core=off
      settings: xl_area=[0, 0, 0, 0, 0, 0, 0]
  Relational : xbsIndex_r3/Relational  mode=a=b  latency=1  explicit_period=off  period=1  en=off  dbl_ovrd=off  show_param=off
      settings: xl_area=[0, 0, 0, 0, 0, 0, 0]
  Slice : xbsIndex_r3/Slice  mode=Lower Bit Location + Width  nbits=1  bit1=0  base1=MSB of Input  bit0=0  base0=LSB of Input  boolean_output=off  explicit_period=off  period=1  dbl_ovrd=off
  fftsync_in : xps_library/gpio  Tag=xps:gpio  io_group=BEE2_usr:rightlink  io_dir=in  arith_type=Boolean  bitwidth=1  bin_pt=0  bit_index=73  sample_period=1  use_single_ended=off  use_ddr=off  reg_iob=on  reg_clk_phase=270  termination=None
  sync_mux : xbsIndex_r3/Mux  inputs=2  precision=Full  arith_type="Signed  (2's comp)"  n_bits=8  bin_pt=2  quantization=Truncate  overflow=Wrap  latency=2  explicit_period=on  period=1  en=off  dbl_ovrd=off  show_param=off  mux_type=off  use_rpm=off  gen_core=off
      settings: xl_area=[0, 0, 0, 0, 0, 0, 0]
  sync_per : xps_library/software register  Tag=xps:sw_reg  io_dir=From Processor  arith_type=Unsigned  bitwidth=32  bin_pt=0  sample_period=1  gw_name=t_t_200_tge5_sync_fft_mux_sync_per_user_data_out
  sync_sel : xps_library/software register  Tag=xps:sw_reg  io_dir=From Processor  arith_type=Unsigned  bitwidth=32  bin_pt=0  sample_period=1  gw_name=t_t_200_tge5_sync_fft_mux_sync_sel_user_data_out
  Out1 : Outport
  wires:
  sync_mux/1 -> Out1/1
  Relational/1 -> Counter/1, sync_mux/3
  sync_per/1 -> Relational/1
  Counter/1 -> Relational/2
  fftsync_in/1 -> sync_mux/2
  Slice/1 -> sync_mux/1
  Constant2/1 -> sync_per/1
  Constant1/1 -> fftsync_in/1
  Constant/1 -> sync_sel/1
  sync_sel/1 -> Slice/1
  Constant3/1 -> Counter/2

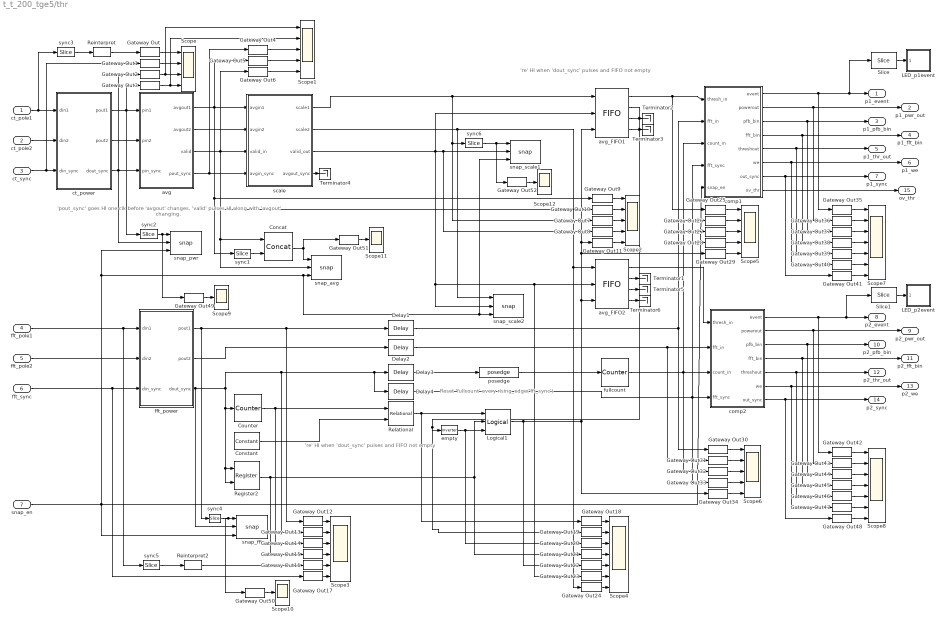
== system t_t_200_tge5/thr ==
  note: 'pout_sync' goes HI one clk
      | before 'avgout' changes.
      | 'valid' pulses HI along with
      | 'avgout' changing.
  note: 're' HI when 'dout_sync'
      | pulses and FIFO not empty
  note: 're' HI when 'dout_sync'
      | pulses and FIFO not empty
  note: Reset 'fullcount' every rising_edge('fft_sync')
  ct_pole1 : Inport  Port=1  LatchInput=off
  ct_pole2 : Inport  Port=2  LatchInput=off
  ct_sync : Inport  Port=3  LatchInput=off
  fft_pole1 : Inport  Port=4  LatchInput=off
  fft_pole2 : Inport  Port=5  LatchInput=off
  fft_sync : Inport  Port=6  LatchInput=off
  "snap_en " : Inport  Port=7  LatchInput=off
  Concat : xbsIndex_r3/Concat  num_inputs=2  explicit_period=off  period=1  dbl_ovrd=off
  Constant : xbsIndex_r3/Constant  const=0  equ=P=C  arith_type=Unsigned  n_bits=FFTSize  bin_pt=0  opselect=C  inp2=PCIN>>17  opr=+  inp1=P  carry=CIN  iostate=0  explicit_period=off  period=1  dbl_ovrd=off
  Counter : xbsIndex_r3/Counter  cnt_type=Free Running  n_bits=FFTSize  bin_pt=0  arith_type=Unsigned  start_count=0  cnt_to=Inf  cnt_by_val=1  operation=Up  explicit_period=off  period=1  load_pin=off  rst=on  en=off  dbl_ovrd=off  show_param=off  use_rpm=on  gen_core=off
      settings: xl_area=[0, 0, 0, 0, 0, 0, 0]
  Delay1 : xbsIndex_r3/Delay  latency=2  reg_retiming=off  explicit_period=off  period=1  en=off  accept_only_valid=off  init_zero=on  dbl_ovrd=off  show_param=off
      settings: xl_area=[0, 0, 0, 0, 0, 0, 0]
  Delay2 : xbsIndex_r3/Delay  latency=2  reg_retiming=off  explicit_period=off  period=1  en=off  accept_only_valid=off  init_zero=on  dbl_ovrd=off  show_param=off
      settings: xl_area=[0, 0, 0, 0, 0, 0, 0]
  Delay3 : xbsIndex_r3/Delay  latency=1  reg_retiming=off  explicit_period=off  period=1  en=off  accept_only_valid=off  init_zero=on  dbl_ovrd=off  show_param=off
      settings: xl_area=[0, 0, 0, 0, 0, 0, 0]
  Delay4 : xbsIndex_r3/Delay  latency=2  reg_retiming=off  explicit_period=off  period=1  en=off  accept_only_valid=off  init_zero=on  dbl_ovrd=off  show_param=off
      settings: xl_area=[0, 0, 0, 0, 0, 0, 0]
  Gateway Out{,1..52} (53 alike) : xbsIndex_r3/Gateway Out  output_type=Double  nbits=8  bin_pt=6  arith_type=Boolean  quantization=Truncate  overflow=Wrap  hdl_port=off  timing_constraint=None  locs_specified=off  LOCs={}  needs_fixed_name=off  show_param=off
      settings: xl_area=[0, 0, 0, 0, 0, 0, 0]
  LED_p1event : Subsystem  mask{pulse_length=200000}
      mask prompts: pulse_length "Pulse Length (samples)"
  LED_p2event : Subsystem  mask{pulse_length=200000}
      mask prompts: pulse_length "Pulse Length (samples)"
  Logical1 : xbsIndex_r3/Logical  logical_function=AND  inputs=3  precision=Full  arith_type=Unsigned  n_bits=8  bin_pt=2  align_bp=on  latency=0  explicit_period=off  period=1  en=off  dbl_ovrd=off  show_param=off
      settings: xl_area=[0, 0, 0, 0, 0, 0, 0]
  Register2 : xbsIndex_r3/Register  init=0  reg_only_valid=off  explicit_period=off  period=1  rst=off  en=on  out_en=off  dbl_ovrd=off  show_param=off
      settings: xl_area=[0, 0, 0, 0, 0, 0, 0]
  Reinterpret : xbsIndex_r3/Reinterpret  force_arith_type=on  arith_type="Signed  (2's comp)"  force_bin_pt=on  bin_pt=DataWidth-1  force_valid=on
  Reinterpret2 : xbsIndex_r3/Reinterpret  force_arith_type=on  arith_type="Signed  (2's comp)"  force_bin_pt=on  bin_pt=DataWidth-1  force_valid=on
  Relational : xbsIndex_r3/Relational  mode=a=b  latency=1  explicit_period=off  period=1  en=off  dbl_ovrd=off  show_param=off
      settings: xl_area=[0, 0, 0, 0, 0, 0, 0]
  Scope : Scope  NumInputPorts=4
      settings: YMin=-5~-5~-5~-5  YMax=5~5~5~5  SaveName=ScopeData9
  Scope{1..2,5..6} (4 alike) : Scope  NumInputPorts=5
      Scope1 settings: YMin=-5~-5~-5~-5~-5  YMax=5~5~5~5~5  SaveName=ScopeData10
      Scope2 settings: TimeRange=4300  YMin=-5~-5~-5~-5~-5  YMax=5~5~5~5~5  SaveName=ScopeData12
      Scope5 settings: YMin=-5~-5~-5~-5~-5  YMax=5~5~5~5~5  SaveName=ScopeData15
      Scope6 settings: YMin=-5~-5~-5~-5~-5  YMax=5~5~5~5~5  SaveName=ScopeData16
  Scope{9..12} (4 alike) : Scope
      Scope10 settings: YMin=8.97459e+008  YMax=9.91929e+008  SaveName=ScopeData23
      Scope11 settings: YMin=8.97459e+008  YMax=9.91929e+008  SaveName=ScopeData24
      Scope12 settings: YMin=8.97459e+008  YMax=9.91929e+008  SaveName=ScopeData25
      Scope9 settings: YMin=9.44694e+008  YMax=9.44694e+008  SaveName=ScopeData22
  Scope3 : Scope  NumInputPorts=6
      settings: YMin=-5~-5~-5~-5~-5~-5  YMax=5~5~5~5~5~5  SaveName=ScopeData13
  Scope4 : Scope  NumInputPorts=7
      settings: YMin=-5~-5~-5~-5~-5~-5~-5  YMax=5~5~5~5~5~5~5  SaveName=ScopeData14
  Scope7 : Scope  NumInputPorts=7
      settings: YMin=0~0~-1~0~0~0~0  YMax=1~1~1~1250~0.5~1~1  SaveName=ScopeData17
  Scope8 : Scope  NumInputPorts=7
      settings: YMin=-5~-5~-5~-5~-5~-5~-5  YMax=5~5~5~5~5~5~5  SaveName=ScopeData18
  Slice : xbsIndex_r3/Slice  mode=Lower Bit Location + Width  nbits=1  bit1=0  base1=MSB of Input  bit0=0  base0=LSB of Input  boolean_output=on  explicit_period=off  period=1  dbl_ovrd=off
  Slice1 : xbsIndex_r3/Slice  mode=Lower Bit Location + Width  nbits=1  bit1=0  base1=MSB of Input  bit0=0  base0=LSB of Input  boolean_output=on  explicit_period=off  period=1  dbl_ovrd=off
  Terminator{1..6} (6 alike) : Terminator
  avg : Subsystem  mask{FFTSize=FFTSize, DataWidth=DataWidth}
      mask prompts: FFTSize "FFT Size (2^?)"; DataWidth "Data Bitwidth"
  avg_FIFO1 : xbsIndex_r3/FIFO  depth=32  percent_nbits=1  store_only_valid=on  init_zero=on  explicit_period=off  period=1  rst=off  en=off  use_almost_empty=off  almost_empty_offset=6  use_almost_full=off  almost_full_offset=6  dbl_ovrd=off  show_param=off  mem_type=Block RAM  gen_core=off
      settings: xl_area=[0, 0, 0, 0, 0, 0, 0]
  avg_FIFO2 : xbsIndex_r3/FIFO  depth=32  percent_nbits=1  store_only_valid=on  init_zero=on  explicit_period=off  period=1  rst=off  en=off  use_almost_empty=off  almost_empty_offset=6  use_almost_full=off  almost_full_offset=6  dbl_ovrd=off  show_param=off  mem_type=Block RAM  gen_core=off
      settings: xl_area=[0, 0, 0, 0, 0, 0, 0]
  comp1 : Subsystem  mask{CPUWidth=CPUWidth, FFTSize=FFTSize, PFBSize=PFBSize}
      mask prompts: CPUWidth "CPU Bitwidth"; FFTSize "FFT Size (2^?)"; PFBSize "PFB Size  (2^?)"
  comp2 : Subsystem  mask{CPUWidth=CPUWidth, FFTSize=FFTSize, PFBSize=PFBSize}
      mask prompts: CPUWidth "CPU Bitwidth"; FFTSize "FFT Size (2^?)"; PFBSize "PFB Size  (2^?)"
  ct_power : Subsystem  mask{mult_lat=3, add_lat=2, DataWidth=DataWidth}
      mask prompts: mult_lat "Multiply Latency"; add_lat "Add Latency"; DataWidth "Data Width"
  empty : xbsIndex_r3/Inverter  latency=0  explicit_period=on  period=1  en=off  dbl_ovrd=off  show_param=off
      settings: xl_area=[0, 0, 0, 0, 0, 0, 0]
  fft_power : Subsystem  mask{mult_lat=3, add_lat=2, DataWidth=DataWidth}
      mask prompts: mult_lat "Multiply Latency"; add_lat "Add Latency"; DataWidth "Data Width"
  fullcount : xbsIndex_r3/Counter  cnt_type=Free Running  n_bits=FFTSize+PFBSize  bin_pt=0  arith_type=Unsigned  start_count=0  cnt_to=Inf  cnt_by_val=1  operation=Up  explicit_period=off  period=1  load_pin=off  rst=on  en=off  dbl_ovrd=off  show_param=off  use_rpm=on  gen_core=off
      settings: xl_area=[0, 0, 0, 0, 0, 0, 0]
  posedge : casper_library/Misc/posedge  Tag=Rising Edge Detector
  scale : Subsystem  mask{DataWidth=DataWidth, mult_lat=4, scale=1}
      mask prompts: DataWidth "Data Bitwidth"; mult_lat "Mulitply Latency"; scale "Test Scale"
  snap_avg : casper_library/Scopes/snap  nsamples=11
  snap_fft : casper_library/Scopes/snap  nsamples=11
  snap_pwr : casper_library/Scopes/snap  nsamples=11
  snap_scale1 : casper_library/Scopes/snap  nsamples=11
  snap_scale2 : casper_library/Scopes/snap  nsamples=11
  sync1 : xbsIndex_r3/Slice  mode=Lower Bit Location + Width  nbits=31  bit1=0  base1=MSB of Input  bit0=0  base0=LSB of Input  boolean_output=off  explicit_period=off  period=1  dbl_ovrd=off
  sync2 : xbsIndex_r3/Slice  mode=Lower Bit Location + Width  nbits=32  bit1=0  base1=MSB of Input  bit0=0  base0=LSB of Input  boolean_output=off  explicit_period=off  period=1  dbl_ovrd=off
  sync3 : xbsIndex_r3/Slice  mode=Lower Bit Location + Width  nbits=DataWidth  bit1=0  base1=MSB of Input  bit0=0  base0=LSB of Input  boolean_output=off  explicit_period=off  period=1  dbl_ovrd=off
  sync4 : xbsIndex_r3/Slice  mode=Lower Bit Location + Width  nbits=DataWidth  bit1=0  base1=MSB of Input  bit0=0  base0=LSB of Input  boolean_output=off  explicit_period=off  period=1  dbl_ovrd=off
  sync5 : xbsIndex_r3/Slice  mode=Lower Bit Location + Width  nbits=DataWidth  bit1=0  base1=MSB of Input  bit0=0  base0=LSB of Input  boolean_output=off  explicit_period=off  period=1  dbl_ovrd=off
  sync6 : xbsIndex_r3/Slice  mode=Lower Bit Location + Width  nbits=32  bit1=0  base1=MSB of Input  bit0=0  base0=LSB of Input  boolean_output=off  explicit_period=off  period=1  dbl_ovrd=off
  p1_event : Outport
  p1_pwr_out : Outport  Port=2
  p1_pfb_bin : Outport  Port=3
  p1_fft_bin : Outport  Port=4
  p1_thr_out : Outport  Port=5
  p1_we : Outport  Port=6
  p1_sync : Outport  Port=7
  p2_event : Outport  Port=8
  p2_pwr_out : Outport  Port=9
  p2_pfb_bin : Outport  Port=10
  p2_fft_bin : Outport  Port=11
  p2_thr_out : Outport  Port=12
  p2_we : Outport  Port=13
  p2_sync : Outport  Port=14
  ov_thr : Outport  Port=15
  wires:
  Slice1/1 -> LED_p2event/1(Sync_In)
  Gateway Out48/1 -> Scope8/7
  Gateway Out47/1 -> Scope8/6
  Gateway Out46/1 -> Scope8/5
  Gateway Out45/1 -> Scope8/4
  Gateway Out44/1 -> Scope8/3
  Gateway Out43/1 -> Scope8/2
  Gateway Out42/1 -> Scope8/1
  Gateway Out41/1 -> Scope7/7
  Gateway Out40/1 -> Scope7/6
  Gateway Out39/1 -> Scope7/5
  Gateway Out38/1 -> Scope7/4
  Gateway Out37/1 -> Scope7/3
  Gateway Out36/1 -> Scope7/2
  Gateway Out35/1 -> Scope7/1
  Gateway Out34/1 -> Scope6/5
  Gateway Out33/1 -> Scope6/4
  Gateway Out32/1 -> Scope6/3
  Gateway Out31/1 -> Scope6/2
  Gateway Out30/1 -> Scope6/1
  Gateway Out29/1 -> Scope5/5
  Gateway Out28/1 -> Scope5/4
  Gateway Out27/1 -> Scope5/3
  Gateway Out26/1 -> Scope5/2
  Gateway Out25/1 -> Scope5/1
  Gateway Out24/1 -> Scope4/7
  Gateway Out23/1 -> Scope4/6
  Gateway Out22/1 -> Scope4/5
  Gateway Out21/1 -> Scope4/4
  Gateway Out20/1 -> Scope4/3
  Gateway Out19/1 -> Scope4/2
  Gateway Out18/1 -> Scope4/1
  Gateway Out17/1 -> Scope3/6
  Gateway Out16/1 -> Scope3/5
  Gateway Out15/1 -> Scope3/4
  Gateway Out14/1 -> Scope3/3
  Gateway Out13/1 -> Scope3/2
  Gateway Out12/1 -> Scope3/1
  Gateway Out11/1 -> Scope2/5
  Gateway Out8/1 -> Scope2/4
  Gateway Out7/1 -> Scope2/3
  Gateway Out10/1 -> Scope2/2
  Gateway Out9/1 -> Scope2/1
  Gateway Out4/1 -> Scope1/3
  Gateway Out5/1 -> Scope1/4
  Gateway Out6/1 -> Scope1/5
  Gateway Out3/1 -> Scope/4, Scope1/2
  Gateway Out2/1 -> Scope/3, Scope1/1
  Gateway Out1/1 -> Scope/2
  Gateway Out/1 -> Scope/1
  Reinterpret/1 -> Gateway Out/1
  sync3/1 -> Reinterpret/1
  ct_sync/1 -> Gateway Out1/1, ct_power/3(din_sync)
  scale/1(scale1) -> Gateway Out7/1, sync6/1, avg_FIFO1/1
  sync2/1 -> snap_pwr/1, Gateway Out49/1
  comp1/6(we) -> p1_we/1, Gateway Out40/1
  comp1/1(event) -> Gateway Out35/1, Slice/1, p1_event/1
  sync1/1 -> Concat/2
  Concat/1 -> snap_avg/1, Gateway Out51/1
  "snap_en "/1 -> snap_pwr/3, snap_avg/3, snap_scale2/3, snap_scale1/3, comp1/5("snap_en "), snap_fft/3
  scale/4(avgout_sync) -> Terminator4/1
  empty/1 -> Gateway Out20/1, Logical1/3
  Logical1/1 -> Gateway Out22/1, Gateway Out34/1, Gateway Out29/1, Gateway Out11/1, avg_FIFO1/3, avg_FIFO2/3
  avg_FIFO1/2 -> Gateway Out19/1, empty/1
  avg/4(pout_sync) -> Gateway Out4/1, scale/4(avgin_sync)
  Delay2/1 -> comp2/2(fft_in), Gateway Out31/1
  Slice/1 -> LED_p1event/1(Sync_In)
  avg/3(valid) -> Gateway Out10/1, Concat/1, snap_avg/2, Gateway Out6/1, scale/3(valid_in)
  Relational/1 -> Gateway Out18/1, Logical1/1
  Register2/1 -> Gateway Out21/1, Logical1/2, Gateway Out15/1
  fft_sync/1 -> Gateway Out17/1, fft_power/3(din_sync)
  fft_pole2/1 -> fft_power/2(din2)
  fft_pole1/1 -> fft_power/1(din1), sync5/1
  ct_pole2/1 -> ct_power/2(din2)
  ct_pole1/1 -> sync3/1, ct_power/1(din1)
  comp2/7(out_sync) -> Gateway Out48/1, p2_sync/1
  comp2/6(we) -> Gateway Out47/1, p2_we/1
  comp2/5(threshout) -> Gateway Out46/1, p2_thr_out/1
  comp2/4(fft_bin) -> Gateway Out45/1, p2_fft_bin/1
  comp2/3(pfb_bin) -> Gateway Out44/1, p2_pfb_bin/1
  comp2/2(powerout) -> Gateway Out43/1, p2_pwr_out/1
  comp2/1(event) -> Slice1/1, p2_event/1, Gateway Out42/1
  comp1/7(out_sync) -> Gateway Out41/1, p1_sync/1
  comp1/5(threshout) -> Gateway Out39/1, p1_thr_out/1
  comp1/4(fft_bin) -> Gateway Out38/1, p1_fft_bin/1
  comp1/3(pfb_bin) -> Gateway Out37/1, p1_pfb_bin/1
  comp1/2(powerout) -> Gateway Out36/1, p1_pwr_out/1
  Delay1/1 -> Gateway Out30/1, Gateway Out26/1, comp1/2(fft_in)
  fullcount/1 -> comp2/3(count_in), Gateway Out32/1, Gateway Out27/1, comp1/3(count_in)
  fft_power/2(pout2) -> Delay2/1
  avg_FIFO2/4 -> Terminator6/1
  avg_FIFO2/3 -> Terminator5/1
  avg_FIFO1/4 -> Terminator3/1
  avg_FIFO1/3 -> Terminator2/1
  avg_FIFO2/1 -> comp2/1(thresh_in)
  fft_power/1(pout1) -> Gateway Out12/1, Delay1/1, sync4/1
  avg_FIFO1/1 -> Gateway Out25/1, comp1/1(thresh_in)
  fft_power/3(dout_sync) -> Gateway Out13/1, Delay3/1, Delay4/1, Counter/1, Register2/1, Register2/2, snap_fft/2
  Constant/1 -> Relational/2
  Counter/1 -> Gateway Out14/1, Relational/1
  scale/3(valid_out) -> Gateway Out8/1, snap_scale1/2, avg_FIFO1/2, Gateway Out23/1, avg_FIFO2/2, snap_scale2/2
  scale/2(scale2) -> Gateway Out24/1, avg_FIFO2/1, snap_scale2/1
  avg/2(avgout2) -> scale/2(avgin2)
  avg/1(avgout1) -> Gateway Out9/1, sync1/1, Gateway Out5/1, scale/1(avgin1)
  ct_power/3(dout_sync) -> Gateway Out2/1, avg/3(pin_sync), snap_pwr/2
  ct_power/2(pout2) -> avg/2(pin2)
  ct_power/1(pout1) -> Gateway Out3/1, sync2/1, avg/1(pin1)
  sync5/1 -> Reinterpret2/1
  Reinterpret2/1 -> Gateway Out16/1
  Delay3/1 -> posedge/1
  posedge/1 -> fullcount/1
  Delay4/1 -> comp2/4(fft_sync), Gateway Out33/1, comp1/4(fft_sync), Gateway Out28/1
  Gateway Out49/1 -> Scope9/1
  sync4/1 -> snap_fft/1, Gateway Out50/1
  Gateway Out50/1 -> Scope10/1
  Gateway Out51/1 -> Scope11/1
  sync6/1 -> snap_scale1/1, Gateway Out52/1
  Gateway Out52/1 -> Scope12/1
  comp1/8(ov_thr) -> ov_thr/1
  avg_FIFO2/2 -> Terminator1/1

== system t_t_200_tge5/ct_in_mux/concat ==
  In1 : Inport  Orientation=down  Port=1  LatchInput=off
  Concat : xbsIndex_r3/Concat  num_inputs=4  explicit_period=on  period=1  dbl_ovrd=off
  Constant : xbsIndex_r3/Constant  const=0  equ=P=C  arith_type=Unsigned  n_bits=14  bin_pt=0  opselect=C  inp2=PCIN>>17  opr=+  inp1=P  carry=CIN  iostate=0  explicit_period=on  period=1  dbl_ovrd=off
  Slice3 : xbsIndex_r3/Slice  mode=Upper Bit Location + Width  nbits=18  bit1=0  base1=MSB of Input  bit0=0  base0=LSB of Input  boolean_output=off  explicit_period=off  period=1  dbl_ovrd=off
  Slice4 : xbsIndex_r3/Slice  mode=Lower Bit Location + Width  nbits=18  bit1=0  base1=MSB of Input  bit0=0  base0=LSB of Input  boolean_output=off  explicit_period=off  period=1  dbl_ovrd=off
  Out1 : Outport
  wires:
  Slice3/1 -> Concat/2
  Constant/1 -> Concat/1, Concat/3
  Slice4/1 -> Concat/4
  In1/1 -> Slice3/1, Slice4/1
  Concat/1 -> Out1/1

== system t_t_200_tge5/ct_in_mux/trig_delay ==
  data_in : Inport  Port=1  LatchInput=off
  trig_in : Inport  Port=2  LatchInput=off
  delay : Inport  Port=3  LatchInput=off
  Constant : xbsIndex_r3/Constant  const=1  equ=P=C  arith_type=Boolean  n_bits=32  bin_pt=0  opselect=C  inp2=PCIN>>17  opr=+  inp1=P  carry=CIN  iostate=0  explicit_period=on  period=1  dbl_ovrd=off
  Counter : xbsIndex_r3/Counter  cnt_type=Free Running  n_bits=32  bin_pt=0  arith_type=Unsigned  start_count=0  cnt_to=Inf  cnt_by_val=1  operation=Up  explicit_period=on  period=1  load_pin=off  rst=on  en=on  dbl_ovrd=off  show_param=off  use_rpm=on  gen_core=off
      settings: xl_area=[0, 0, 0, 0, 0, 0, 0]
  Delay : xbsIndex_r3/Delay  latency=2  reg_retiming=off  explicit_period=on  period=1  en=off  accept_only_valid=off  init_zero=on  dbl_ovrd=off  show_param=off
      settings: xl_area=[0, 0, 0, 0, 0, 0, 0]
  Gateway Out : xbsIndex_r3/Gateway Out  output_type=Double  nbits=8  bin_pt=6  arith_type=Boolean  quantization=Truncate  overflow=Wrap  hdl_port=on  timing_constraint=None  locs_specified=off  LOCs={}  needs_fixed_name=off  show_param=off
      settings: xl_area=[0, 0, 0, 0, 0, 0, 0]
  Gateway Out1 : xbsIndex_r3/Gateway Out  output_type=Double  nbits=8  bin_pt=6  arith_type=Boolean  quantization=Truncate  overflow=Wrap  hdl_port=on  timing_constraint=None  locs_specified=off  LOCs={}  needs_fixed_name=off  show_param=off
      settings: xl_area=[0, 0, 0, 0, 0, 0, 0]
  Register : xbsIndex_r3/Register  init=0  reg_only_valid=off  explicit_period=on  period=1  rst=on  en=on  out_en=off  dbl_ovrd=off  show_param=off
      settings: xl_area=[0, 0, 0, 0, 0, 0, 0]
  Relational : xbsIndex_r3/Relational  mode=a=b  latency=1  explicit_period=on  period=1  en=on  dbl_ovrd=off  show_param=off
      settings: xl_area=[0, 0, 0, 0, 0, 0, 0]
  Scope : Scope  NumInputPorts=2
      settings: YMin=-5~-5  YMax=5~5
  posedge : casper_library/Misc/posedge  Tag=Rising Edge Detector
  data_out : Outport
  trig_out : Outport  Port=2
  wires:
  delay/1 -> Relational/1
  trig_in/1 -> Register/3, Gateway Out1/1
  Constant/1 -> Register/1
  Relational/1 -> Register/2, Counter/1, Gateway Out/1, posedge/1
  Register/1 -> Counter/2, Relational/3
  Counter/1 -> Relational/2
  Gateway Out/1 -> Scope/1
  Gateway Out1/1 -> Scope/2
  data_in/1 -> Delay/1
  Delay/1 -> data_out/1
  posedge/1 -> trig_out/1
